simulink model "swevomotor2"  (R2024b)
settings: Solver=VariableStepAuto  StartTime=0.0  StopTime=10.0  RelTol=1e-3
model workspace (MAT data in the model file):
  J = 5e-05
  K = 0.2
  L = 0.01
  R = 4
  V = 7.4
  b = 0.0005
  ki = 7
  kp = 9
  ts = 0.01
libraries: SignalEditorBlockLib x1
settings Model: Creator=jigya  LastModifiedBy=jigya

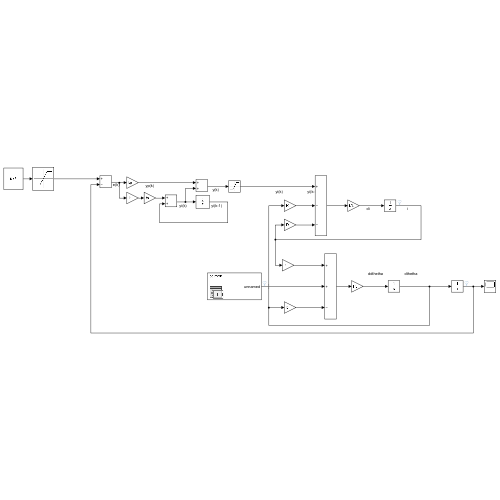
[thumbnail: Simulink's stored preview of the top-level diagram]
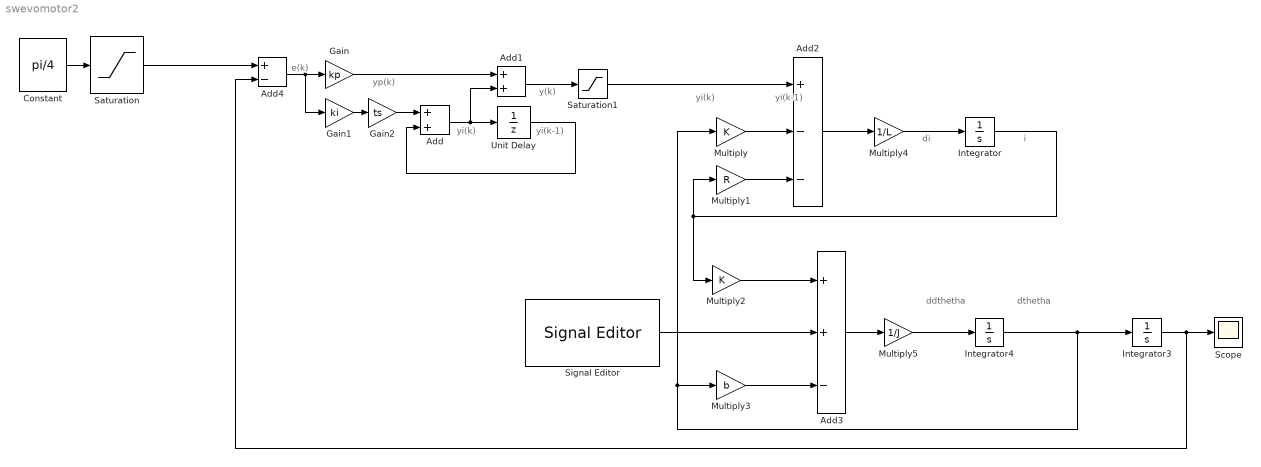
== system swevomotor2 ==
  note: di
  note: dthetha
  note: ddthetha
  note: i
  note: yi(k-1)
  note: yi(k)
  note: yi(k-1)
  note: e(k)
  note: yp(k)
  note: yi(k)
  note: y(k)
  Add : Sum
  Add1 : Sum
  Add2 : Sum  Inputs=+--
  Add3 : Sum  Inputs=++-
  Add4 : Sum  Inputs=+-
  Constant : Constant  Value=pi/4
  Gain : Gain  Gain=kp
  Gain1 : Gain  Gain=ki
  Gain2 : Gain  Gain=ts
  Integrator : Integrator
  Integrator3 : Integrator
  Integrator4 : Integrator
  Multiply : Gain  Gain=K
  Multiply1 : Gain  Gain=R
  Multiply2 : Gain  Gain=K
  Multiply3 : Gain  Gain=b
  Multiply4 : Gain  Gain=1/L
  Multiply5 : Gain  Gain=1/J
  Saturation : Saturate
  Saturation1 : Saturate
  Scope : Scope
  Signal Editor : SignalEditorBlockLib/Signal Editor  FileName=disturbance.mat  ActiveScenario=calmAir  ActiveSignal=unnamed  IsBus=off  OutputBusObjectStr=Bus: BusObject  SampleTime=0  Interpolate=off  ZeroCross=off  OutputAfterFinalValue=Setting to zero  Unit=inherit  PreserveSignalName=on  ApplySigPropsToAllScenarios=on  ApplySigPropsToAllSignals=off
  Unit Delay : UnitDelay  SampleTime=-1  HasFrameUpgradeWarning=on
  wires:
  Multiply4/1 -> Integrator/1
  Add2/1 -> Multiply4/1
  Multiply2/1 -> Add3/1
  Multiply/1 -> Add2/2
  Saturation1/1 -> Add2/1
  Integrator/1 -> Multiply1/1, Multiply2/1
  Add3/1 -> Multiply5/1
  Multiply5/1 -> Integrator4/1
  Multiply1/1 -> Add2/3
  Integrator4/1 -> Integrator3/1, Multiply/1, Multiply3/1
  Multiply3/1 -> Add3/3
  Gain2/1 -> Add/1
  Gain1/1 -> Gain2/1
  Integrator3/1 -> Add4/2, Scope/1
  Add/1 -> Unit Delay/1, Add1/2
  Add1/1 -> Saturation1/1
  Gain/1 -> Add1/1
  Unit Delay/1 -> Add/2
  Add4/1 -> Gain/1, Gain1/1
  Saturation/1 -> Add4/1
  Constant/1 -> Saturation/1
  Signal Editor/1 -> Add3/2
